simulink model "Ex7"  (R2019a)
settings: Solver=VariableStepAuto  StartTime=0.0  StopTime=40
settings Model: Creator=toshi  LastModifiedBy=toshi
settings SolverCC: MaxConsecutiveZCs=10000

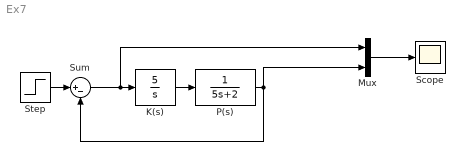
== system Ex7 ==
  K(s) : TransferFcn  Numerator=[5]  Denominator=[1 0]
  Mux : Mux  Inputs=2
  P(s) : TransferFcn  Denominator=[5 2]
  Scope : Scope
  Step : Step  Time=0  SampleTime=0.01
  Sum : Sum  Inputs=|+-
  wires:
  P(s)/1 -> Mux/2, Sum/2
  K(s)/1 -> P(s)/1
  Step/1 -> Sum/1
  Sum/1 -> Mux/1, K(s)/1
  Mux/1 -> Scope/1
